simulink model "State_Flow_v0"  (R2013a)
settings: Solver=ode5  StartTime=0.0  StopTime=20  RelTol=1e-3
undefined symbols (not defined in the file or in its folder): magnitude
libraries: simulink x2
settings Model: SimulationMode=external  CovModelRefEnable=off  Creator=Arnav  LastModifiedBy=s4358046
settings DataIOCC: LimitDataPoints=off  SaveFormat=StructureWithTime
settings DebuggingCC: UnderspecifiedInitializationDetection=Simplified  MergeDetectMultiDrivingBlocksExec=error  SolverPrmCheckMsg=none  FrameProcessingCompatibilityMsg=error  StateNameClashWarn=none
settings HardwareCC: ProdIntDivRoundTo=Zero  ProdEndianess=LittleEndian  ProdHWDeviceType=Generic->32-bit x86 compatible  TargetIntDivRoundTo=Zero  TargetEndianess=LittleEndian  TargetHWDeviceType=MATLAB Host  ProdEqTarget=off
settings ModelReferenceCC: PropagateSignalLabelsOutOfModel=on
settings RTWCC: SystemTargetFile=rtwin.tlc  TemplateMakefile=rtwin.tmf  Description=Real-Time Windows Target  ProcessScript=rtwin_make_rtw_hook  RTWCompilerOptimization=On
settings CodeAppCC: MaxIdLength=95
settings RTWinTargetCC: TargetLibSuffix=_rtwin.lib  TargetPreCompLibLocation=C:\Program Files\MATLAB\R2013a\toolbox\rtw\targets\rtwin\lib\win64  CodeReplacementLibrary=ANSI_C  RTWinDir=C:/PROGRA~1/MATLAB/R2013a/toolbox/rtw/targets/rtwin  TargetArch=win64

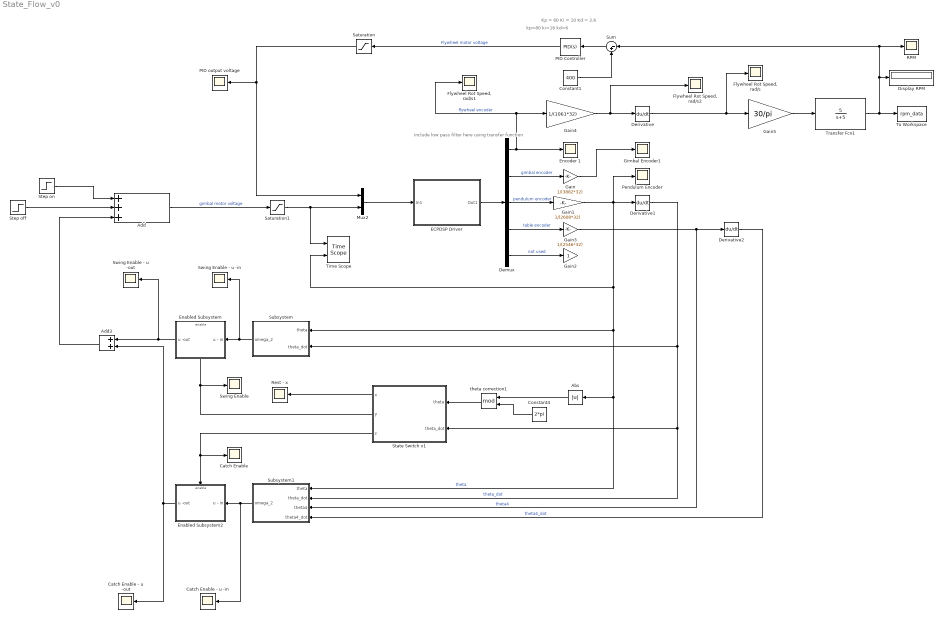
== system State_Flow_v0 ==
  note: Kp = 60
      | Ki = 10
      | Kd = 2.6
  note: include low pass filter here
      | using transfer function
  note: kp=80
      | ki=16
      | kd=6
  Abs : Abs
  Add : Sum  Inputs=+++
  Add3 : Sum
  Catch Enable : Scope
      settings: YMin=-10  YMax=10  SaveName=ScopeData3
  Catch Enable - u -in : Scope
      settings: YMin=-10  YMax=10  SaveName=ScopeData4
  Catch Enable - u -out : Scope
      settings: YMin=-10  YMax=10  SaveName=ScopeData5
  Constant1 : Constant  Value=400
  Constant4 : Constant  Value=2*pi
  Demux : Demux  Outputs=5
  Derivative : Derivative
  Derivative1 : Derivative
  Derivative2 : Derivative
  Display RPM : Display
  ECPDSP Driver : Subsystem  mask{BaseAddr='0xC000', STime=0.008, TimeOutPer=500, HWAccess=on}
      mask prompts: BaseAddr "Base I/O Address"; STime "Sample Time (Sec)"; TimeOutPer "Timeout Period (500 ~ 2000)"; HWAccess "Hardware Access"
      mask Display: color('black');disp('ECPDSP Driver\n upto\n 4 Encs(ADC Channels)\n and 2 Dacs')
  Enabled Subsystem : Subsystem  TreatAsAtomicUnit=on
  Enabled Subsystem2 : Subsystem  TreatAsAtomicUnit=on
  Encoder 1 : Scope
      settings: YMin=1.5e+06  YMax=8.5e+06  SaveName=ScopeData12
  "Flywheel Rot Speed, rad/s" : Scope
      settings: YMin=-10  YMax=10  SaveName=ScopeData13
  "Flywheel Rot Speed, rad/s1" : Scope
      settings: YMin=-10  YMax=10  SaveName=ScopeData14
  "Flywheel Rot Speed, rad/s2" : Scope
      settings: YMin=-10  YMax=10  SaveName=ScopeData15
  Gain : Gain  Gain=1/(3882*32)
  Gain1 : Gain  Gain=1/(2608*32)
  Gain2 : Gain
  Gain3 : Gain  Gain=1/(2546*32)
  Gain4 : Gain  Gain=1/(1061*32)
  Gain5 : Gain  Gain=30/pi
  Gimbal Encoder1 : Scope
      settings: YMin=-0.25  YMax=3.25  SaveName=ScopeData9
  Mux2 : Mux  Inputs=2
  PID Controller : simulink/Continuous/PID Controller  Controller=PID  TimeDomain=Continuous-time  SampleTime=-1  IntegratorMethod=Forward Euler  FilterMethod=Forward Euler  Form=Parallel  P=60  I=10  D=2.6  N=100  InitialConditionSource=internal  InitialConditionForIntegrator=0  InitialConditionForFilter=0  ExternalReset=none  LimitOutput=off  UpperSaturationLimit=inf  LowerSaturationLimit=-inf  LinearizeAsGain=on  AntiWindupMode=none  Kb=1  TrackingMode=off  Kt=1  PParamMin=[]  PParamMax=[]  IParamMin=[]  IParamMax=[]  DParamMin=[]  DParamMax=[]  NParamMin=[]  NParamMax=[]  KbParamMin=[]  KbParamMax=[]  KtParamMin=[]  KtParamMax=[]  POutMin=[]  POutMax=[]  IOutMin=[]  IOutMax=[]  DOutMin=[]  DOutMax=[]  NOutMin=[]  NOutMax=[]  KbOutMin=[]  KbOutMax=[]  KtOutMin=[]  KtOutMax=[]  IntegratorOutMin=[]  IntegratorOutMax=[]  FilterOutMin=[]  FilterOutMax=[]  SumOutMin=[]  SumOutMax=[]  SumI1OutMin=[]  SumI1OutMax=[]  SumI2OutMin=[]  SumI2OutMax=[]  SumI3OutMin=[]  SumI3OutMax=[]  SumDOutMin=[]  SumDOutMax=[]  SaturationOutMin=[]  SaturationOutMax=[]  IntegratorContinuousStateAttributes=''  IntegratorStateMustResolveToSignalObject=off  IntegratorRTWStateStorageClass=Auto  FilterContinuousStateAttributes=''  FilterStateMustResolveToSignalObject=off  FilterRTWStateStorageClass=Auto
  PID output voltage : Scope
      settings: YMin=400  YMax=421  SaveName=ScopeData6
  Pendulum Encoder : Scope
      settings: YMin=-0.25  YMax=3.25  SaveName=ScopeData16
  RPM : Scope
      settings: YMin=400  YMax=421  SaveName=ScopeData17
  Rest - x : Scope
      settings: YMin=-10  YMax=10  SaveName=ScopeData19
  Saturation : Saturate  UpperLimit=32000  LowerLimit=-32000
  Saturation1 : Saturate  UpperLimit=22000  LowerLimit=-22000
  State Switch v1 : Stateflow chart  TreatAsAtomicUnit=on
  Step off : Step  Time=30.15  After=-14000  SampleTime=0
  Step on : Step  Time=30  After=14000  SampleTime=0
  Subsystem : Subsystem
  Subsystem1 : Subsystem
  Sum : Sum  Inputs=|-+
  Swing Enable : Scope
      settings: YMin=-10  YMax=10  SaveName=ScopeData2
  Swing Enable - u -in : Scope
      settings: YMin=-10  YMax=10
  Swing Enable - u -out : Scope
      settings: YMin=-10  YMax=10
  Time Scope : TimeScope  NumInputPorts=2  DefaultConfigurationName=spbscopes.TimeScopeBlockCfg
      settings: CopyFcn=scopeextensions.ScopeBlock.callback(gcbh, 'onBlockCopy', gcbh);  DeleteFcn=scopeextensions.ScopeBlock.callback(gcbh, 'onBlockDelete');  PreSaveFcn=scopeextensions.ScopeBlock.callback(gcbh, 'onModelSave');  NameChangeFcn=scopeextensions.ScopeBlock.callback(gcbh, 'onBlockRename');  CloseFcn=scopeextensions.ScopeBlock.callback(gcbh, 'onBlockClose');  PreDeleteFcn=scopeextensions.ScopeBlock.callback(gcbh, 'onBlockPreDelete');
  To Workspace : ToWorkspace  VariableName=rpm_data  SampleTime=-1  SaveFormat=Timeseries
  Transfer Fcn1 : TransferFcn  Numerator=[5]  Denominator=[1 5]
  theta correction1 : Math  Operator=mod  SaturateOnIntegerOverflow=on
  wires:
  ECPDSP Driver/1(Out1) -> Demux/1
  Demux/1 -> Encoder 1/1, Gain4/1, "Flywheel Rot Speed, rad/s1"/1  "flywheel encoder"
  PID Controller/1 -> Saturation/1  "Flywheel motor voltage"
  Demux/2 -> Gain/1  "gimbal encoder"
  Demux/3 -> Gain1/1  "pendulum encoder"
  Demux/4 -> Gain3/1  "table encoder"
  Demux/5 -> Gain2/1  "not used"
  Gain4/1 -> "Flywheel Rot Speed, rad/s2"/1, Derivative/1
  Constant1/1 -> Sum/2
  Sum/1 -> PID Controller/1
  Saturation/1 -> PID output voltage/1, Mux2/1
  Derivative/1 -> Gain5/1, "Flywheel Rot Speed, rad/s"/1
  Gain5/1 -> Transfer Fcn1/1
  Step off/1 -> Add/2
  Step on/1 -> Add/1
  Add/1 -> Saturation1/1  "gimbal motor voltage"
  Derivative1/1 -> Subsystem/2(theta_dot), Subsystem1/2(theta_dot), State Switch v1/2(theta_dot)  "theta_dot"
  Add3/1 -> Add/3
  Saturation1/1 -> Time Scope/1, Mux2/2
  Mux2/1 -> ECPDSP Driver/1(In1)
  Gain/1 -> Gimbal Encoder1/1
  Transfer Fcn1/1 -> To Workspace/1, Display RPM/1, RPM/1, Sum/1
  State Switch v1/1(x) -> Rest - x/1
  theta correction1/1 -> State Switch v1/1(theta)
  Constant4/1 -> theta correction1/2
  Gain1/1 -> Time Scope/2, Subsystem/1(theta), Subsystem1/1(theta), Abs/1, Derivative1/1, Pendulum Encoder/1  "theta"
  State Switch v1/2(y) -> Swing Enable/1, Enabled Subsystem/Enable
  State Switch v1/3(z) -> Catch Enable/1, Enabled Subsystem2/Enable
  Subsystem/1(omega_2) -> Enabled Subsystem/1(u - in), Swing Enable - u -in/1
  Enabled Subsystem/1(u -out) -> Swing Enable - u -out/1, Add3/1
  Gain3/1 -> Subsystem1/3(theta4), Derivative2/1  "theta4"
  Derivative2/1 -> Subsystem1/4(theta4_dot)  "theta4_dot"
  Abs/1 -> theta correction1/1
  Subsystem1/1(omega_2) -> Catch Enable - u -in/1, Enabled Subsystem2/1(u - in)
  Enabled Subsystem2/1(u -out) -> Catch Enable - u -out/1, Add3/2

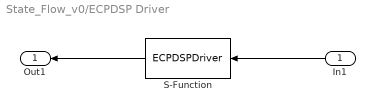
== system State_Flow_v0/ECPDSP Driver ==
  In1 : Inport
  S-Function : S-Function  FunctionName=ECPDSPDriver  Parameters=BaseAddr,STime,TimeOutPer,HWAccess  EnableBusSupport=off
  Out1 : Outport
  wires:
  In1/1 -> S-Function/1
  S-Function/1 -> Out1/1

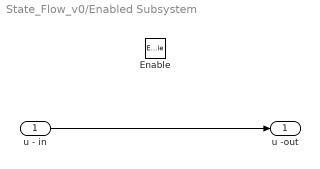
== system State_Flow_v0/Enabled Subsystem ==
  u - in : Inport
  Enable : EnablePort
  u -out : Outport  InitialOutput=[0]
  wires:
  u - in/1 -> u -out/1

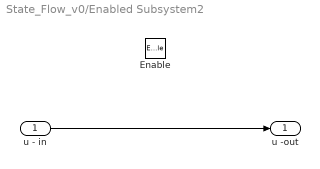
== system State_Flow_v0/Enabled Subsystem2 ==
  u - in : Inport
  Enable : EnablePort
  u -out : Outport  InitialOutput=[0]
  wires:
  u - in/1 -> u -out/1

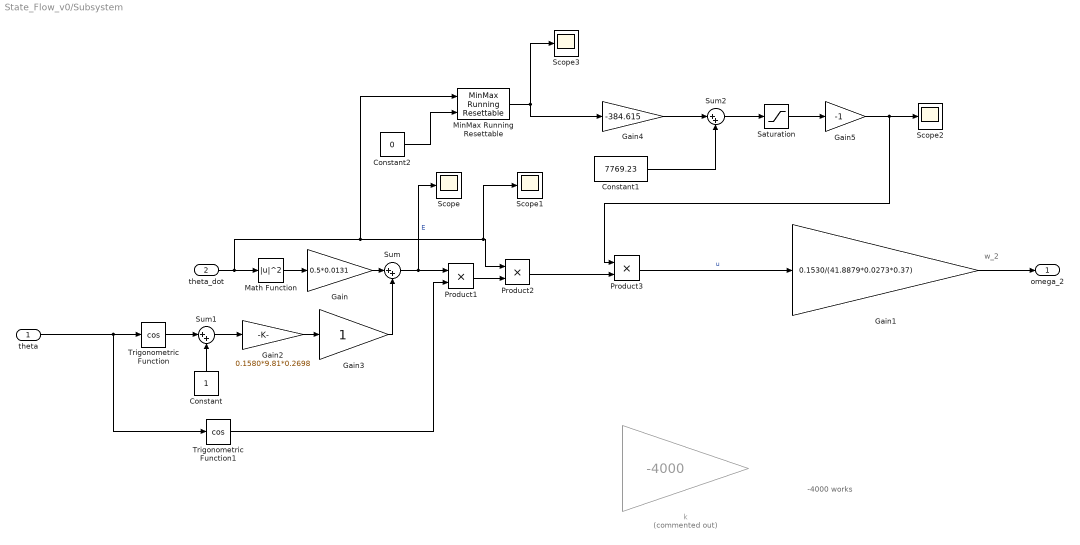
== system State_Flow_v0/Subsystem ==
  note: -4000 works
  note: w_2
  theta : Inport
  theta_dot : Inport  Port=2
  Constant : Constant
  Constant1 : Constant  Value=7769.23
  Constant2 : Constant  Value=0
  Gain : Gain  Gain=0.5*0.0131
  Gain1 : Gain  Gain=0.1530/(41.8879*0.0273*0.37)
  Gain2 : Gain  Gain=0.1580*9.81*0.2698
  Gain3 : Gain
  Gain4 : Gain  Gain=-384.615
  Gain5 : Gain  Gain=-1
  Math Function : Math  Operator=magnitude^2  SaturateOnIntegerOverflow=on
  MinMax Running Resettable : simulink/Math Operations/MinMax Running Resettable  Function=max  vinit=0.0
  Product1 : Product
  Product2 : Product
  Product3 : Product
  Saturation : Saturate  UpperLimit=7000  LowerLimit=2000
  Scope{,1..3} (4 alike) : Scope
      Scope settings: YMin=-10  YMax=10  SaveName=ScopeData7
      Scope1 settings: YMin=-10  YMax=10  SaveName=ScopeData8
      Scope2 settings: YMin=-10  YMax=10  SaveName=ScopeData10
      Scope3 settings: YMin=-10  YMax=10  SaveName=ScopeData11
  Sum : Sum  Inputs=|++
  Sum1 : Sum  Inputs=|++
  Sum2 : Sum  Inputs=|++
  Trigonometric Function : Trigonometry  Operator=cos
  Trigonometric Function1 : Trigonometry  Operator=cos
  k : Gain  Commented=on  Gain=-4000
  omega_2 : Outport
  wires:
  theta_dot/1 -> MinMax Running Resettable/1, Scope1/1, Product2/1, Math Function/1
  Math Function/1 -> Gain/1
  Gain/1 -> Sum/1
  Product3/1 -> Gain1/1  "u"
  Gain1/1 -> omega_2/1
  Trigonometric Function/1 -> Sum1/1
  Constant/1 -> Sum1/2
  Sum1/1 -> Gain2/1
  Gain2/1 -> Gain3/1
  Sum/1 -> Product1/1, Scope/1  "E"
  Trigonometric Function1/1 -> Product1/2
  Product1/1 -> Product2/2
  Product2/1 -> Product3/2
  theta/1 -> Trigonometric Function1/1, Trigonometric Function/1
  Gain3/1 -> Sum/2
  MinMax Running Resettable/1 -> Gain4/1, Scope3/1
  Gain4/1 -> Sum2/1
  Constant1/1 -> Sum2/2
  Sum2/1 -> Saturation/1
  Saturation/1 -> Gain5/1
  Gain5/1 -> Product3/1, Scope2/1
  Constant2/1 -> MinMax Running Resettable/2

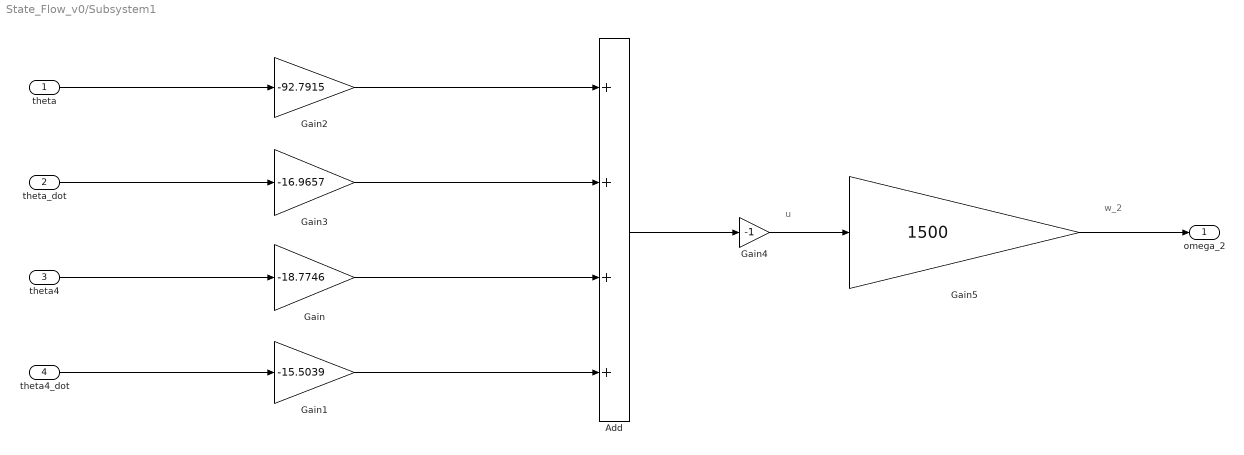
== system State_Flow_v0/Subsystem1 ==
  note: w_2
  note: u
  theta : Inport
  theta_dot : Inport  Port=2
  theta4 : Inport  Port=3
  theta4_dot : Inport  Port=4
  Add : Sum  Inputs=++++
  Gain : Gain  Gain=-18.7746
  Gain1 : Gain  Gain=-15.5039
  Gain2 : Gain  Gain=-92.7915
  Gain3 : Gain  Gain=-16.9657
  Gain4 : Gain  Gain=-1
  Gain5 : Gain  Gain=1500
  omega_2 : Outport
  wires:
  Add/1 -> Gain4/1
  Gain2/1 -> Add/1
  Gain3/1 -> Add/2
  theta/1 -> Gain2/1
  theta_dot/1 -> Gain3/1
  Gain/1 -> Add/3
  Gain1/1 -> Add/4
  theta4/1 -> Gain/1
  theta4_dot/1 -> Gain1/1
  Gain5/1 -> omega_2/1
  Gain4/1 -> Gain5/1

== stateflow chart State_Flow_v0/State Switch v1 ==
  state Swing
    entry:
    x = 0,
    y = 1,
    z = 0;
  state Rest
    entry:
    x = 1,
    y = 0,
    z = 0;
  state Catch
    entry:
    x = 0,
    y = 0,
    z = 1;
  (default) -> Rest
  Rest -> Swing : [theta > 0.05 & theta_dot > 0.05]
  Swing -> Rest [order 2] : [theta < 0.05 & theta_dot < 0.05]
  Swing -> Catch [order 1] : [(3.14 - (3.14/8)) < theta & theta < (3.14 + (3.14/8))]
  Catch -> Swing : [theta < (3.14 - (3.14/8)) | theta > (3.14 + (3.14/8))]
  data: x output; y output; z output; theta input; theta_dot input
